simulink model "roboticArm_loadCell"  (R2021a)
settings: Solver=FixedStepDiscrete  StartTime=0.0  StopTime=inf  FixedStep=0.001  RelTol=1e-3  EnableMultiTasking=on
PreLoadFcn:
  | init_roboticArm_loadCell();
values from neighbouring files (symbols this model uses):
  Kd_matr = zeros(6)    [initRoboticArm.m]    (also in init_roboticArm_loadCell.m = diag([0.00;0;0.003;0.0001;0.00;0.0001]); zeroForce2.mat = [0 0 0 0 0 0 0 0 0 0 0 0 ... (36 elements, 6x6)])
  Ki_matr = zeros(6)    [initRoboticArm.m]    (also in init_roboticArm_loadCell.m = diag([10;100;10;30;10;2]); zeroForce2.mat = [10 0 0 0 0 0 0 100 0 0 0 0 ... (36 elements, 6x6)])
  Kp_matr = zeros(6)    [initRoboticArm.m]    (also in init_roboticArm_loadCell.m = diag([0.3;0.1;0.2;0.05;0.3;0.2]); zeroForce2.mat = [0.3 0 0 0 0 0 0 0.1 0 0 0 0 ... (36 elements, 6x6)])
  scaled_array = zeros(round((chirp_duration+10)*1./dt-1)+1,7)    [initRoboticArm.m]    (also in init_roboticArm_loadCell.m = [scaled_array(:,1) zeros(length(scaled_array),6)]; scaled_array_oc5.mat = [0 0.0141421356237 0.0282842712475 0.0424264068712 0.0565685; zeroForce2.mat = [0 0.0141421356237 0.0282842712475 0.0424264068712 0.0565685)
undefined symbols (not defined in the file or in its folder): DiscIntNeverNeededParam
libraries: franka_simulink_library x5, franka_simulink_library_misc x4, etargetslib x2, simulink x2, dspnetwork x2
settings Model: SimulationMode=external  ExtModeTrigDuration=1000000  Creator=vasi_ko  LastModifiedBy=host
settings SolverCC: AlgebraicLoopSolver=TrustRegion
settings DataIOCC: LimitDataPoints=on  SaveFormat=Array  ReturnWorkspaceOutputs=off
settings OptimizationCC: DefaultParameterBehavior=Inlined  EnhancedBackFolding=on  PassReuseOutputArgsAs=Individual arguments  ZeroExternalMemoryAtStartup=off  ZeroInternalMemoryAtStartup=off  OptimizeBlockOrder=speed  DifferentSizesBufferReuse=on  OptimizationCustomize=off  EfficientTunableParamExpr=on
settings DebuggingCC: SolverPrmCheckMsg=warning  ParameterTunabilityLossMsg=error  SFUnexpectedBacktrackingDiag=warning  SFNoUnconditionalDefaultTransitionDiag=warning  SFExecutionAtInitializationDiag=none  SFMachineParentedDataDiag=warning  ArithmeticOperatorsInVariantConditions=warning
settings HardwareCC: ProdBitPerLong=64  ProdHWDeviceType=Intel->x86-64 (Linux 64)
settings ModelReferenceCC: PropagateSignalLabelsOutOfModel=off
settings SFSimCC: SimUseLocalCustomCode=off  MATLABDynamicMemAlloc=off  CustomCodeUndefinedFunction=UseInterfaceOnly  SimTargetLang=C++
settings RTWCC: SystemTargetFile=franka_emika_panda.tlc  GenCodeOnly=on  TemplateMakefile=ert_default_tmf  RTWVerbose=off  RTWUseLocalCustomCode=off  Toolchain=Franka Simulink | gmake (64-bit linux)  BuildConfiguration=Specify  IncludeHyperlinkInReport=on  TargetLang=C++
settings CodeAppCC: ForceParamTrailComments=on  IgnoreCustomStorageClasses=off  OperatorAnnotations=on  SimulinkDataObjDesc=on  SFDataObjDesc=on  InsertBlockDesc=on
settings STFCustomTargetCC: TargetLangStandard=C99 (ISO)  MultiwordLength=256  GenerateSampleERTMain=on  ModelReferenceCompliant=off  CombineOutputUpdateFcns=on  ERTCustomFileBanners=on  SupportNonInlinedSFcns=off  RemoveResetFunc=on  MATLABClassNameForMDSCustomization=Simulink.SoftwareTarget.ERTCustomization  CPPClassGenCompliant=on  GRTInterface=off  SystemTargetFile=franka_emika_panda.tlc
settings ERTTargetCC: TargetLangStandard=C99 (ISO)  GenerateSampleERTMain=on  ModelReferenceCompliant=off  ParMdlRefBuildCompliant=off  CompOptLevelCompliant=off  ConcurrentExecutionCompliant=off  SupportContinuousTime=on  ModelStepFunctionPrototypeControlCompliant=off  ExtMode=on  ExtModeMexArgs='10.10.10.11' 0 17725  InlinedParameterPlacement=NonHierarchical  ERTCustomFileTemplate=franka_emika_panda_file_process.tlc
settings ConfigComp: CovMetricSettings=dw  CovSaveCumulativeToWorkspaceVar=on  CovSaveSingleToWorkspaceVar=on  CovExternalEMLEnable=off  CovSFcnEnable=off

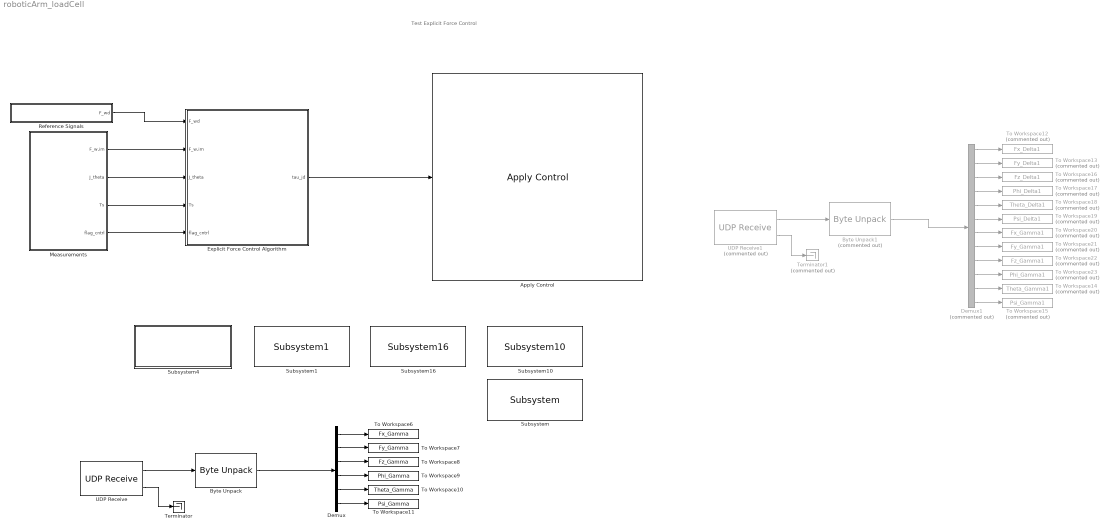
== system roboticArm_loadCell ==
  note: Test Explicit Force Control
  Apply Control : franka_simulink_library/Apply Control  robot_ip=robot_ip  gripper_attached=off  control_mode=Torque Control  controller_choice=Joint Impedance Controller  elbow_control=on  collision_thresholds=100*ones(1,52)  joint_impedance=joint_impedance  cartesian_impedance=cartesian_impedance  load_inertia=load_inertia  EE_T_K=EE_T_K  init_joint_configuration_req=off  init_joint_configuration=[0.00392584915725334;-0.104076810189763;0.0404703493577216;-2.7334242600631;0.0113035300040543;2.63364770337236;0.372162046953987]
      settings: SourceProductName=Franka Emika
  Byte Unpack : etargetslib/Byte Unpack  dimensions={[6]}  datatypes={'double'}  byteAlign=1
  Byte Unpack1 : etargetslib/Byte Unpack  Commented=on  dimensions={[12]}  datatypes={'double'}  byteAlign=1
  Demux : Demux  Outputs=6
  Demux1 : Demux  Commented=on  Outputs=12
  Explicit Force Control Algorithm : Subsystem
  Measurements : Subsystem
  Reference Signals : Subsystem
  Subsystem : franka_simulink_library_misc/Subsystem  SystemSampleTime=-1  VariantActivationTime=update diagram  Latency=0  AutoFrameSizeCalculation=off
  Subsystem1 : franka_simulink_library_misc/Subsystem1  SystemSampleTime=-1  VariantActivationTime=update diagram  Latency=0  AutoFrameSizeCalculation=off
  Subsystem10 : franka_simulink_library_misc/Subsystem10  SystemSampleTime=-1  VariantActivationTime=update diagram  Latency=0  AutoFrameSizeCalculation=off
  Subsystem16 : franka_simulink_library_misc/Subsystem16  SystemSampleTime=-1  VariantActivationTime=update diagram  Latency=0  AutoFrameSizeCalculation=off
  Subsystem4 : Subsystem  AncestorBlock=franka_simulink_library_misc/Subsystem4
      settings: OpenFcn=|
      | model_name = fileparts(gcb);
      | 
      | %set_up_franka_simulink_model( model_name, 'external_mode_on' );
      | build_standalone(model_name,'-DON_TARGET_WAIT_FOR_START=1');
      mask Display: fprintf('Generate code with External Mode on\n & Build standalone executable\n\n Double click on me!');
  Terminator : Terminator
  Terminator1 : Terminator  Commented=on
  To Workspace10 : ToWorkspace  VariableName=Theta_Gamma  SaveFormat=Structure With Time  SampleTime=-1
  To Workspace11 : ToWorkspace  VariableName=Psi_Gamma  SaveFormat=Structure With Time  SampleTime=-1
  To Workspace12 : ToWorkspace  Commented=on  VariableName=Fx_Delta1  SaveFormat=Structure With Time  SampleTime=-1
  To Workspace13 : ToWorkspace  Commented=on  VariableName=Fy_Delta1  SaveFormat=Structure With Time  SampleTime=-1
  To Workspace14 : ToWorkspace  Commented=on  VariableName=Theta_Gamma1  SaveFormat=Structure With Time  SampleTime=-1
  To Workspace15 : ToWorkspace  Commented=on  VariableName=Psi_Gamma1  SaveFormat=Structure With Time  SampleTime=-1
  To Workspace16 : ToWorkspace  Commented=on  VariableName=Fz_Delta1  SaveFormat=Structure With Time  SampleTime=-1
  To Workspace17 : ToWorkspace  Commented=on  VariableName=Phi_Delta1  SaveFormat=Structure With Time  SampleTime=-1
  To Workspace18 : ToWorkspace  Commented=on  VariableName=Theta_Delta1  SaveFormat=Structure With Time  SampleTime=-1
  To Workspace19 : ToWorkspace  Commented=on  VariableName=Psi_Delta1  SaveFormat=Structure With Time  SampleTime=-1
  To Workspace20 : ToWorkspace  Commented=on  VariableName=Fx_Gamma1  SaveFormat=Structure With Time  SampleTime=-1
  To Workspace21 : ToWorkspace  Commented=on  VariableName=Fy_Gamma1  SaveFormat=Structure With Time  SampleTime=-1
  To Workspace22 : ToWorkspace  Commented=on  VariableName=Fz_Gamma1  SaveFormat=Structure With Time  SampleTime=-1
  To Workspace23 : ToWorkspace  Commented=on  VariableName=Phi_Gamma1  SaveFormat=Structure With Time  SampleTime=-1
  To Workspace6 : ToWorkspace  VariableName=Fx_Gamma  SaveFormat=Structure With Time  SampleTime=-1
  To Workspace7 : ToWorkspace  VariableName=Fy_Gamma  SaveFormat=Structure With Time  SampleTime=-1
  To Workspace8 : ToWorkspace  VariableName=Fz_Gamma  SaveFormat=Structure With Time  SampleTime=-1
  To Workspace9 : ToWorkspace  VariableName=Phi_Gamma  SaveFormat=Structure With Time  SampleTime=-1
  UDP Receive : dspnetwork/UDP Receive  localURL='0.0.0.0'  localPort=8002  remoteURL='10.10.10.15'  remotePort=-1  recvBufferSize=8192  dims=96/2  signalDatatype=uint8  isComplex=off  isVarSize=off  showBlockingTime=on  blockingTime=inf  sampletime=0.001  blockPlatform=HOST
  UDP Receive1 : dspnetwork/UDP Receive  Commented=on  localURL='0.0.0.0'  localPort=8002  remoteURL='10.10.10.15'  remotePort=-1  recvBufferSize=8192  dims=96  signalDatatype=uint8  isComplex=off  isVarSize=off  showBlockingTime=on  blockingTime=inf  sampletime=0.001  blockPlatform=HOST
  wires:
  Explicit Force Control Algorithm/1(tau_jd) -> Apply Control/1
  Measurements/1(F_w,im) -> Explicit Force Control Algorithm/2(F_w,im)
  Measurements/2(J_theta) -> Explicit Force Control Algorithm/3(J_theta)
  Measurements/3(Ts) -> Explicit Force Control Algorithm/4(Ts)
  Measurements/4(flag_cntrl) -> Explicit Force Control Algorithm/5(flag_cntrl)
  Reference Signals/1(F_wd) -> Explicit Force Control Algorithm/1(F_wd)
  Byte Unpack/1 -> Demux/1
  UDP Receive/1 -> Byte Unpack/1
  UDP Receive/2 -> Terminator/1
  Demux/6 -> To Workspace11/1
  Demux/5 -> To Workspace10/1
  Demux/4 -> To Workspace9/1
  Demux/3 -> To Workspace8/1
  Demux/2 -> To Workspace7/1
  Demux/1 -> To Workspace6/1
  Demux1/7 -> To Workspace20/1
  Demux1/8 -> To Workspace21/1
  Demux1/9 -> To Workspace22/1
  Demux1/10 -> To Workspace23/1
  Demux1/11 -> To Workspace14/1
  Demux1/12 -> To Workspace15/1
  Demux1/6 -> To Workspace19/1
  Demux1/5 -> To Workspace18/1
  Demux1/4 -> To Workspace17/1
  Demux1/3 -> To Workspace16/1
  Demux1/2 -> To Workspace13/1
  Demux1/1 -> To Workspace12/1
  UDP Receive1/2 -> Terminator1/1
  UDP Receive1/1 -> Byte Unpack1/1
  Byte Unpack1/1 -> Demux1/1

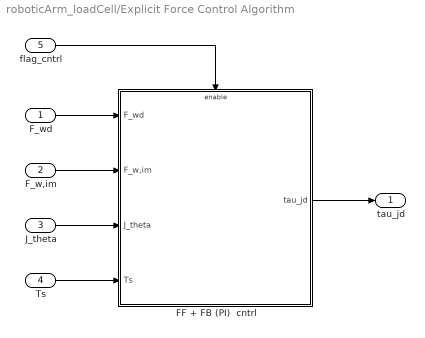
== system roboticArm_loadCell/Explicit Force Control Algorithm ==
  F_wd : Inport
  F_w,im : Inport  Port=2
  J_theta : Inport  Port=3
  Ts : Inport  Port=4
  flag_cntrl : Inport  Port=5
  FF + FB (PI)  cntrl : Subsystem
  tau_jd : Outport
  wires:
  F_wd/1 -> FF + FB (PI)  cntrl/1(F_wd)
  F_w,im/1 -> FF + FB (PI)  cntrl/2(F_w,im)
  J_theta/1 -> FF + FB (PI)  cntrl/3(J_theta)
  Ts/1 -> FF + FB (PI)  cntrl/4(Ts)
  FF + FB (PI)  cntrl/1(tau_jd) -> tau_jd/1
  flag_cntrl/1 -> FF + FB (PI)  cntrl/Enable

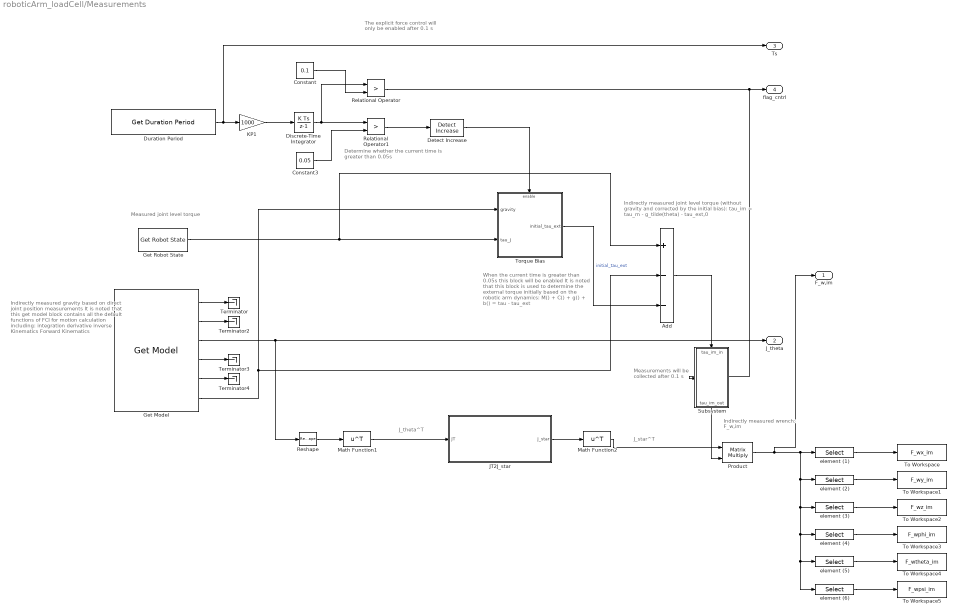
== system roboticArm_loadCell/Measurements ==
  note: Indirectly measured wrench:
      | F_w,im
  note: J_star^T
  note: J_theta^T
  note: The explicit force control will only be enabled after 0.1 s
  note: When the current time is greater than 0.05s this block will be enabled
      |
      | It is noted that this block is used to determine the external torque initially based on the robotic arm dynamics:
      |
      | M() + C() + g() + b() = tau - tau_ext
  note: Determine whether the current time is greater than 0.05s
  note: Measured joint level torque
  note: Indirectly measured gravity based on direct joint position measurements
      |
      | It is noted that this get model block contains all the default functions of FCI for motion calculation including:
      | integration
      | derivative
      | inverse Kinematics
      | Forward Kinematics
  note: Indirectly measured joint level torque (without gravity and corrected by the initial bias):
      | tau_im = tau_m - g_tilde(theta) - tau_ext,0
  note: Measurements will be collected after 0.1 s
  Add : Sum  Inputs=+--
  Constant : Constant  Value=0.1
  Constant3 : Constant  Value=0.05
  Detect Increase : simulink/Logic and Bit Operations/Detect Increase  vinit=0.0  OutDataTypeStr=boolean
  Discrete-Time Integrator : DiscreteIntegrator  SampleTime=-1  ICPrevOutput=DiscIntNeverNeededParam  ICPrevScaledInput=DiscIntNeverNeededParam
  Duration Period : franka_simulink_library/Get Duration Period  robot_ip=robot_ip
      settings: SourceProductName=Franka Emika
  Get Model : franka_simulink_library/Get Model  robot_ip=robot_ip
      settings: SourceProductName=Franka Emika
  Get Robot State : franka_simulink_library/Get Robot State  robot_ip=robot_ip  signals_requested='tau_J'
      settings: SourceProductName=Franka Emika
  JT2J_star : MATLAB Function  TreatAsAtomicUnit=on
  KP1 : Gain  Gain=1000
  Math Function1 : Math  Operator=transpose  SignedPower=on  SaturateOnIntegerOverflow=on
  Math Function2 : Math  Operator=transpose  SignedPower=on  SaturateOnIntegerOverflow=on
  Product : Product  Multiplication=Matrix(*)
  Relational Operator : RelationalOperator  Operator=>  OutDataTypeStr=boolean  RndMeth=Nearest
  Relational Operator1 : RelationalOperator  Operator=>  OutDataTypeStr=boolean  RndMeth=Nearest
  Reshape : Reshape  OutputDimensionality=Customize  OutputDimensions=[6,7]
  Subsystem : Subsystem
  Terminator{,2..4} (4 alike) : Terminator
  To Workspace : ToWorkspace  VariableName=F_wx_im  SaveFormat=Structure With Time  SampleTime=-1
  To Workspace1 : ToWorkspace  VariableName=F_wy_im  SaveFormat=Structure With Time  SampleTime=-1
  To Workspace2 : ToWorkspace  VariableName=F_wz_im  SaveFormat=Structure With Time  SampleTime=-1
  To Workspace3 : ToWorkspace  VariableName=F_wphi_im  SaveFormat=Structure With Time  SampleTime=-1
  To Workspace4 : ToWorkspace  VariableName=F_wtheta_im  SaveFormat=Structure With Time  SampleTime=-1
  To Workspace5 : ToWorkspace  VariableName=F_wpsi_im  SaveFormat=Structure With Time  SampleTime=-1
  Torque Bias : Subsystem
  element (1) : Selector  InputPortWidth=6  IndexOptions=Index vector (dialog)  Indices=1  OutputSizes=1
  element (2) : Selector  InputPortWidth=6  IndexOptions=Index vector (dialog)  Indices=2  OutputSizes=1
  element (3) : Selector  InputPortWidth=6  IndexOptions=Index vector (dialog)  Indices=3  OutputSizes=1
  element (4) : Selector  InputPortWidth=6  IndexOptions=Index vector (dialog)  Indices=4  OutputSizes=1
  element (5) : Selector  InputPortWidth=6  IndexOptions=Index vector (dialog)  Indices=5  OutputSizes=1
  element (6) : Selector  InputPortWidth=6  IndexOptions=Index vector (dialog)  Indices=6  OutputSizes=1
  F_w,im : Outport
  J_theta : Outport  Port=2
  Ts : Outport  Port=3
  flag_cntrl : Outport  Port=4
  wires:
  Relational Operator1/1 -> Detect Increase/1
  Duration Period/1 -> Ts/1, KP1/1
  Constant3/1 -> Relational Operator1/2
  Discrete-Time Integrator/1 -> Relational Operator/1, Relational Operator1/1
  KP1/1 -> Discrete-Time Integrator/1
  Detect Increase/1 -> Torque Bias/Enable
  Get Robot State/1 -> Add/1, Torque Bias/2(tau_J)
  Get Model/6 -> Add/2, Torque Bias/1(gravity)
  Get Model/1 -> Terminator/1
  Get Model/2 -> Terminator2/1
  Get Model/4 -> Terminator3/1
  Get Model/5 -> Terminator4/1
  Torque Bias/1(initial_tau_ext) -> Add/3  "initial_tau_ext"
  Add/1 -> Subsystem/1(tau_im_in)
  Get Model/3 -> Reshape/1, J_theta/1
  Reshape/1 -> Math Function1/1
  Math Function1/1 -> JT2J_star/1(JT)
  JT2J_star/1(J_star) -> Math Function2/1
  Math Function2/1 -> Product/1
  Product/1 -> F_w,im/1, element (2)/1, element (3)/1, element (6)/1, element (5)/1, element (4)/1, element (1)/1
  element (1)/1 -> To Workspace/1
  element (6)/1 -> To Workspace5/1
  element (5)/1 -> To Workspace4/1
  element (4)/1 -> To Workspace3/1
  element (3)/1 -> To Workspace2/1
  element (2)/1 -> To Workspace1/1
  Constant/1 -> Relational Operator/2
  Relational Operator/1 -> Subsystem/Enable, flag_cntrl/1
  Subsystem/1(tau_im_out) -> Product/2

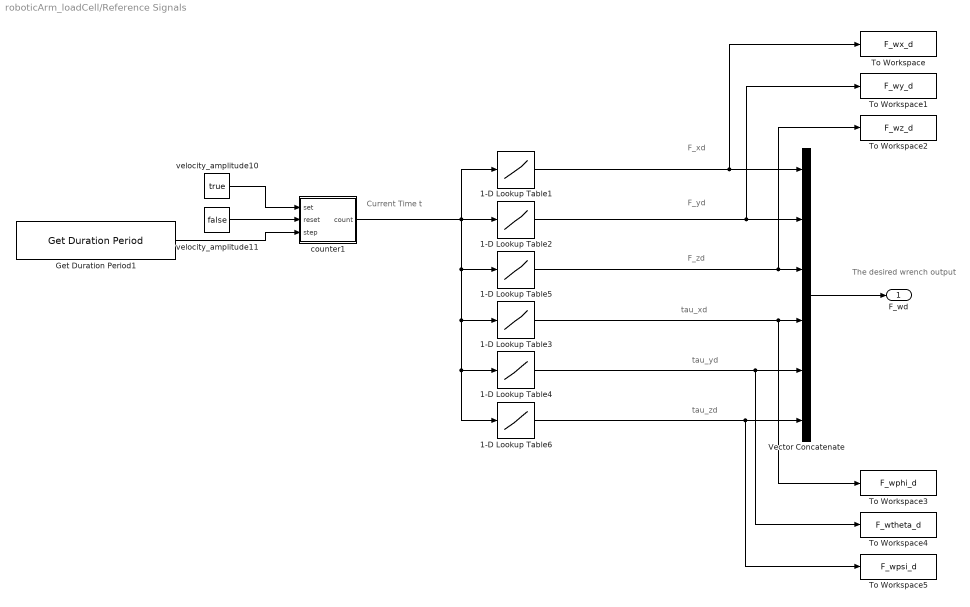
== system roboticArm_loadCell/Reference Signals ==
  note: Current Time t
  note: F_xd
  note: F_yd
  note: F_zd
  note: tau_xd
  note: tau_yd
  note: tau_zd
  note: The desired wrench output
  1-D Lookup Table1 : Lookup_n-D  NumberOfTableDimensions=1  BreakpointsForDimension1=scaled_array(1:10000,1)  Table=scaled_array(1:10000,2)  InternalRulePriority=Speed  RndMeth=Simplest  InputSameDT=on
  1-D Lookup Table2 : Lookup_n-D  NumberOfTableDimensions=1  BreakpointsForDimension1=scaled_array(1:10000,1)  Table=scaled_array(1:10000,3)  InternalRulePriority=Speed  RndMeth=Simplest  InputSameDT=on
  1-D Lookup Table3 : Lookup_n-D  NumberOfTableDimensions=1  BreakpointsForDimension1=scaled_array(1:10000,1)  Table=scaled_array(1:10000,5)  InternalRulePriority=Speed  RndMeth=Simplest  InputSameDT=on
  1-D Lookup Table4 : Lookup_n-D  NumberOfTableDimensions=1  BreakpointsForDimension1=scaled_array(1:10000,1)  Table=scaled_array(1:10000,6)  InternalRulePriority=Speed  RndMeth=Simplest  InputSameDT=on
  1-D Lookup Table5 : Lookup_n-D  NumberOfTableDimensions=1  BreakpointsForDimension1=scaled_array(1:10000,1)  Table=scaled_array(1:10000,4)  InternalRulePriority=Speed  RndMeth=Simplest  InputSameDT=on
  1-D Lookup Table6 : Lookup_n-D  NumberOfTableDimensions=1  BreakpointsForDimension1=scaled_array(1:10000,1)  Table=scaled_array(1:10000,7)  InternalRulePriority=Speed  RndMeth=Simplest  InputSameDT=on
  Get Duration Period1 : franka_simulink_library/Get Duration Period  robot_ip=robot_ip
      settings: SourceProductName=Franka Emika
  To Workspace : ToWorkspace  VariableName=F_wx_d  SaveFormat=Structure With Time  SampleTime=-1
  To Workspace1 : ToWorkspace  VariableName=F_wy_d  SaveFormat=Structure With Time  SampleTime=-1
  To Workspace2 : ToWorkspace  VariableName=F_wz_d  SaveFormat=Structure With Time  SampleTime=-1
  To Workspace3 : ToWorkspace  VariableName=F_wphi_d  SaveFormat=Structure With Time  SampleTime=-1
  To Workspace4 : ToWorkspace  VariableName=F_wtheta_d  SaveFormat=Structure With Time  SampleTime=-1
  To Workspace5 : ToWorkspace  VariableName=F_wpsi_d  SaveFormat=Structure With Time  SampleTime=-1
  Vector Concatenate : Concatenate  NumInputs=6
  counter1 : Subsystem
  velocity_amplitude10 : Constant  Value=true  VectorParams1D=off
  velocity_amplitude11 : Constant  Value=false  VectorParams1D=off
  F_wd : Outport
  wires:
  counter1/1(count) -> 1-D Lookup Table6/1, 1-D Lookup Table4/1, 1-D Lookup Table3/1, 1-D Lookup Table5/1, 1-D Lookup Table2/1, 1-D Lookup Table1/1
  Vector Concatenate/1 -> F_wd/1
  Get Duration Period1/1 -> counter1/3(step)
  velocity_amplitude10/1 -> counter1/1(set)
  velocity_amplitude11/1 -> counter1/2(reset)
  1-D Lookup Table5/1 -> To Workspace2/1, Vector Concatenate/3
  1-D Lookup Table3/1 -> To Workspace3/1, Vector Concatenate/4
  1-D Lookup Table6/1 -> To Workspace5/1, Vector Concatenate/6
  1-D Lookup Table4/1 -> To Workspace4/1, Vector Concatenate/5
  1-D Lookup Table1/1 -> To Workspace/1, Vector Concatenate/1
  1-D Lookup Table2/1 -> To Workspace1/1, Vector Concatenate/2

== system roboticArm_loadCell/Subsystem4 ==

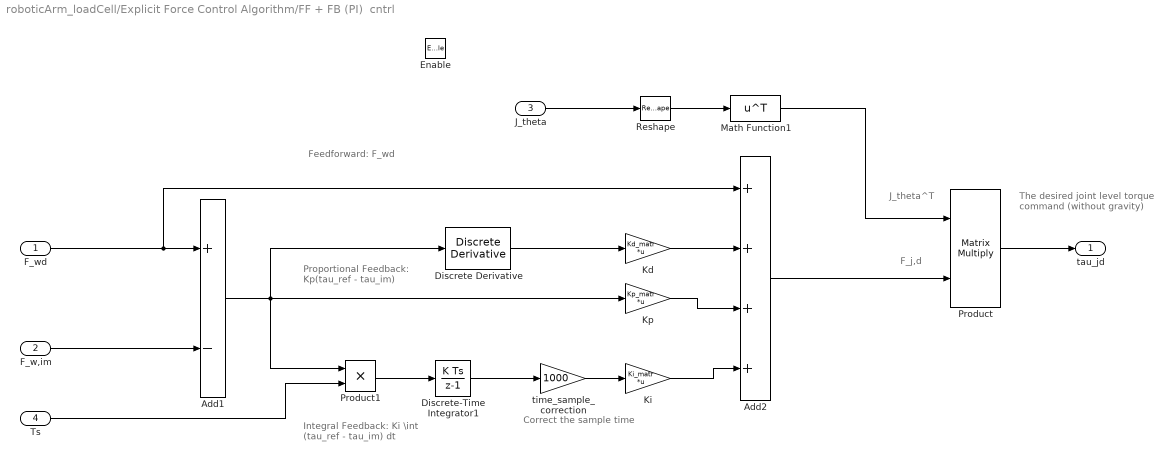
== system roboticArm_loadCell/Explicit Force Control Algorithm/FF + FB (PI)  cntrl ==
  note: F_j,d
  note: The desired joint level torque command (without gravity)
  note: Feedforward:
      | F_wd
  note: Integral Feedback:
      | Ki \int (tau_ref - tau_im) dt
  note: Proportional Feedback:
      |  Kp(tau_ref - tau_im)
  note: Correct the sample time
  note: J_theta^T
  F_wd : Inport
  F_w,im : Inport  Port=2
  J_theta : Inport  Port=3
  Ts : Inport  Port=4
  Enable : EnablePort
  Add1 : Sum  Inputs=+-
  Add2 : Sum  Inputs=++++
  Discrete Derivative : simulink/Discrete/Discrete Derivative  gainval=1.0  ICPrevScaledInput=0.0  OutMin=[]  OutMax=[]  OutDataType=fixdt(1, 16)  OutScaling=2^-10  DoSatur=off
  Discrete-Time Integrator1 : DiscreteIntegrator  SampleTime=0.001  ICPrevOutput=DiscIntNeverNeededParam  ICPrevScaledInput=DiscIntNeverNeededParam
  Kd : Gain  Gain=Kd_matr  Multiplication=Matrix(K*u)
  Ki : Gain  Gain=Ki_matr  Multiplication=Matrix(K*u)
  Kp : Gain  Gain=Kp_matr  Multiplication=Matrix(K*u)
  Math Function1 : Math  Operator=transpose  SignedPower=on  SaturateOnIntegerOverflow=on
  Product : Product  Multiplication=Matrix(*)
  Product1 : Product
  Reshape : Reshape  OutputDimensionality=Customize  OutputDimensions=[6,7]
  time_sample_correction : Gain  Gain=1000
  tau_jd : Outport
  wires:
  Product1/1 -> Discrete-Time Integrator1/1
  Ts/1 -> Product1/2
  F_wd/1 -> Add2/1, Add1/1
  Add1/1 -> Discrete Derivative/1, Product1/1, Kp/1
  Discrete-Time Integrator1/1 -> time_sample_correction/1
  Reshape/1 -> Math Function1/1
  J_theta/1 -> Reshape/1
  Math Function1/1 -> Product/1
  time_sample_correction/1 -> Ki/1
  Discrete Derivative/1 -> Kd/1
  Kp/1 -> Add2/3
  Ki/1 -> Add2/4
  Kd/1 -> Add2/2
  F_w,im/1 -> Add1/2
  Add2/1 -> Product/2
  Product/1 -> tau_jd/1

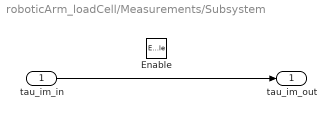
== system roboticArm_loadCell/Measurements/Subsystem ==
  tau_im_in : Inport
  Enable : EnablePort
  tau_im_out : Outport
  wires:
  tau_im_in/1 -> tau_im_out/1

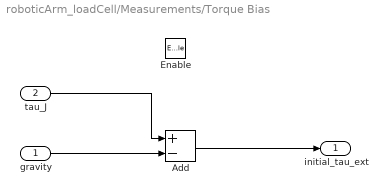
== system roboticArm_loadCell/Measurements/Torque Bias ==
  gravity : Inport
  tau_J : Inport  Port=2
  Enable : EnablePort
  Add : Sum  Inputs=+-
  initial_tau_ext : Outport  InitialOutput=[0 0 0 0 0 0 0]  VectorParamsAs1DForOutWhenUnconnected=off
  wires:
  tau_J/1 -> Add/1
  gravity/1 -> Add/2
  Add/1 -> initial_tau_ext/1

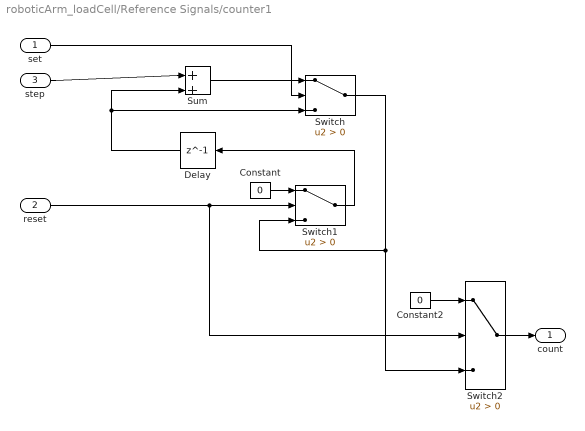
== system roboticArm_loadCell/Reference Signals/counter1 ==
  set : Inport  OutDataTypeStr=boolean
  reset : Inport  Port=2  OutDataTypeStr=boolean
  step : Inport  Port=3  OutDataTypeStr=double
  Constant : Constant  Value=0  OutDataTypeStr=double
  Constant2 : Constant  Value=0  OutDataTypeStr=double
  Delay : Delay  DelayLength=1  InitialCondition=0
  Sum : Sum  Inputs=|++
  Switch : Switch  Criteria=u2 > Threshold
  Switch1 : Switch  Criteria=u2 > Threshold  OutDataTypeStr=double
  Switch2 : Switch  Criteria=u2 > Threshold  OutDataTypeStr=double
  count : Outport  OutDataTypeStr=double  VectorParamsAs1DForOutWhenUnconnected=off
  wires:
  Switch2/1 -> count/1
  Constant2/1 -> Switch2/1
  Sum/1 -> Switch/1
  set/1 -> Switch/2
  Switch/1 -> Switch1/3, Switch2/3
  step/1 -> Sum/1
  Delay/1 -> Sum/2, Switch/3
  reset/1 -> Switch1/2, Switch2/2
  Constant/1 -> Switch1/1
  Switch1/1 -> Delay/1

== matlab function roboticArm_loadCell/Measurements/JT2J_star ==
  data: JT input; J_star output
function J_star = JT2J_star(JT)
%#codegen

J = JT';
% low isotropic damping, the value should be much smaller than lambda_max^2
beta =0;
% damping added in singular directions, we chose it to be equal to
% threshold
% lambda_max = singularity_threshold_inverse_kinematics; 
% SVD decomposition
[U,S,~] = svd(J);
sigma = diag(S);
% rank
singularity_threshold_inverse_kinematics = eps;
r = sum(sigma > singularity_threshold_inverse_kinematics);
% initilizing damping
  lambda_square_vector = zeros(6,1);
if r==6 % damping in full rank case is zero
    lambda_square_vector = zeros(6,1);
else % daamping in rank deficient cases
%     sigma_singular = sigma(r+1:6);
%     lambda_square_vector(r+1:6) = ...
%         (1 - (sigma_singular/ singularity_threshold_inverse_kinematics).^2) *...
%         lambda_max^2;
end
J_star =  JT * U * diag(1./(sigma.^2+lambda_square_vector+beta^2*ones(6,1)))*U';

end
